simulink model "bogliolo_bozzi_simulink"  (R2019a)
settings: Solver=VariableStepAuto  StartTime=0.0  StopTime=10.0  RelTol=1e-3
values from neighbouring files (symbols this model uses):
  k = 2    [bogliolo_bozzi.m]
settings Model: Creator=asus  LastModifiedBy=asus

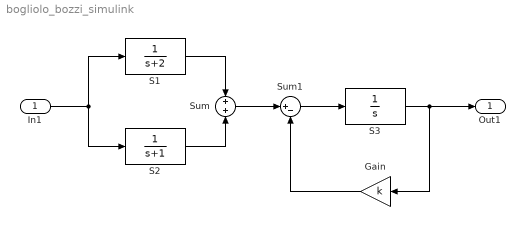
== system bogliolo_bozzi_simulink ==
  In1 : Inport
  " S1" : TransferFcn  Denominator=[1 2]
  Gain : Gain  Gain=k
  S2 : TransferFcn  Denominator=[1 1]
  S3 : TransferFcn  Denominator=[1 0]
  Sum : Sum  Inputs=+|+
  Sum1 : Sum  Inputs=|+-
  Out1 : Outport
  wires:
  In1/1 -> S2/1, " S1"/1
  " S1"/1 -> Sum/1
  S2/1 -> Sum/2
  S3/1 -> Gain/1, Out1/1
  Gain/1 -> Sum1/2
  Sum/1 -> Sum1/1
  Sum1/1 -> S3/1
